simulink model "fig4"  (R2021b)
settings: Solver=VariableStepAuto  StartTime=0.0  StopTime=10.0  RelTol=1e-3
values from neighbouring files (symbols this model uses):
  P = randi(10, [1 length(t)])    [plot_fig8_train_diagram.m]    (also in run_sim_ac.m = fn_get_params_simu(1, N); run_sim_fb1.m = fn_get_params_simu(1, 1); run_sim_fb2.m = P_)
libraries: fuzblock x10
settings Model: Creator=Alex  LastModifiedBy=Alex

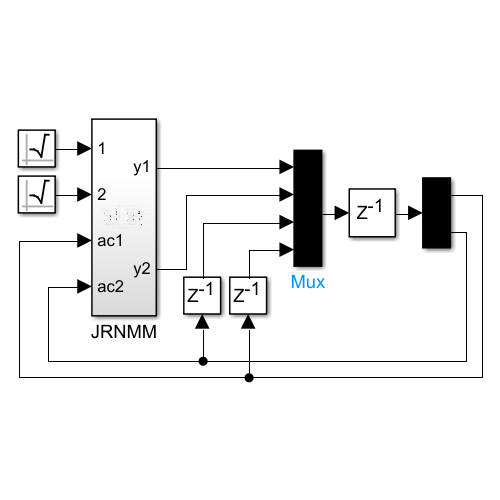
[thumbnail: Simulink's stored preview of the top-level diagram]
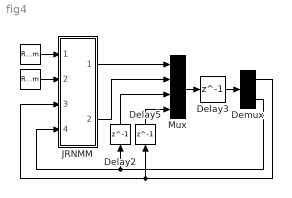
== system fig4 ==
  " " : RandomNumber  Seed=1  SampleTime=0.001
  "  " : RandomNumber  Seed=1  SampleTime=0.001
  Delay2 : Delay  DelayLength=1  InitialCondition=0
  Delay3 : Delay  DelayLength=1  InitialCondition=0
  Delay5 : Delay  DelayLength=1  InitialCondition=0
  Demux : Demux  Outputs=2
  JRNMM : Subsystem
  Mux : Mux
  wires:
  "  "/1 -> JRNMM/1(In2)
  " "/1 -> JRNMM/2(In1)
  JRNMM/1(y1) -> Mux/1
  Demux/1 -> Delay5/1, JRNMM/3(ac1)
  Demux/2 -> JRNMM/4(ac2), Delay2/1
  Mux/1 -> Delay3/1
  Delay3/1 -> Demux/1
  JRNMM/2(y2) -> Mux/2
  Delay2/1 -> Mux/3
  Delay5/1 -> Mux/4

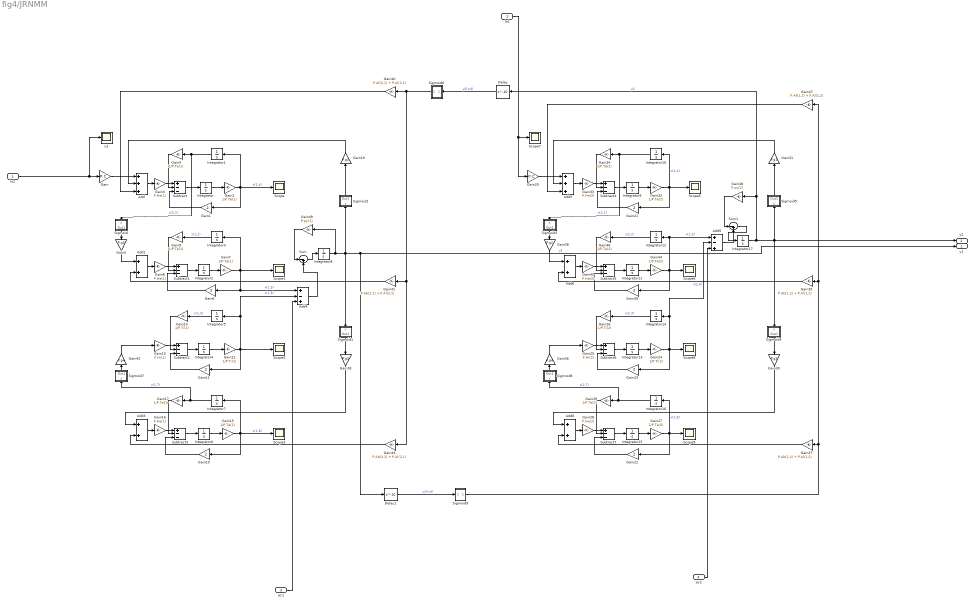
== system fig4/JRNMM ==
  In2 : Inport
  In1 : Inport  Port=2
  ac1 : Inport  Port=3
  ac2 : Inport  Port=4
  Add : Sum  Inputs=+++
  Add{1,3,6,8} (4 alike) : Sum
  Add4 : Sum  Inputs=+-+
  Add5 : Sum  Inputs=+++
  Add9 : Sum  Inputs=+-+
  Delay : Delay  DelayLength=10  InitialCondition=0
  Delay1 : Delay  DelayLength=10  InitialCondition=0  SampleTime=0.-1
  Gain : Gain  Gain=P.C
  Gain{1,6,10..11,21..23,39} (8 alike) : Gain  Gain=2
  Gain12 : Gain  Gain=1/P.Ti(1)
  Gain13 : Gain  Gain=P.Hi(1)
  Gain14 : Gain  Gain=1/P.Ti(1)
  Gain{2,4,7,9,15,17} (6 alike) : Gain  Gain=1/P.Te(1)
  Gain16 : Gain  Gain=P.He(1)
  Gain18 : Gain  Gain=P.g3
  Gain19 : Gain  Gain=P.g1
  Gain20 : Gain  Gain=P.C
  Gain24 : Gain  Gain=1/P.Ti(2)
  Gain25 : Gain  Gain=P.Hi(2)
  Gain26 : Gain  Gain=1/P.Ti(2)
  Gain{27,29,32,34,44,46} (6 alike) : Gain  Gain=1/P.Te(2)
  Gain28 : Gain  Gain=P.He(2)
  Gain3 : Gain  Gain=P.He(1)
  Gain30 : Gain  Gain=P.g3
  Gain31 : Gain  Gain=P.g1
  Gain33 : Gain  Gain=P.He(2)
  Gain35 : Gain  Gain=P.Ab(1,2) + P.Al(1,2)
  Gain36 : Gain  Gain=P.g4
  Gain37 : Gain  Gain=P.Ab(1,2) + P.Al(1,2)
  Gain38 : Gain  Gain=P.g2
  Gain40 : Gain  Gain=P.Af(2,1) + P.Al(2,1)
  Gain41 : Gain  Gain=P.Ab(2,1) + P.Al(2,1)
  Gain42 : Gain  Gain=P.g4
  Gain43 : Gain  Gain=P.Ab(2,1) + P.Al(2,1)
  Gain45 : Gain  Gain=P.He(2)
  Gain47 : Gain  Gain=P.Af(1,2) + P.Al(1,2)
  Gain48 : Gain  Gain=P.py(2)
  Gain49 : Gain  Gain=P.py(1)
  Gain5 : Gain  Gain=P.g2
  Gain8 : Gain  Gain=P.He(1)
  Integrator : Integrator  ContinuousStateAttributes='x14'
  Integrator1 : Integrator  ContinuousStateAttributes='x11'
  Integrator10 : Integrator  ContinuousStateAttributes='x21'
  Integrator11 : Integrator  ContinuousStateAttributes='x25'
  Integrator12 : Integrator  ContinuousStateAttributes='x22'
  Integrator13 : Integrator  ContinuousStateAttributes='x26'
  Integrator14 : Integrator  ContinuousStateAttributes='x23'
  Integrator15 : Integrator  ContinuousStateAttributes='x28'
  Integrator16 : Integrator  ContinuousStateAttributes='x27'
  Integrator17 : Integrator
  Integrator2 : Integrator  ContinuousStateAttributes='x15'
  Integrator3 : Integrator  ContinuousStateAttributes='x12'
  Integrator4 : Integrator  ContinuousStateAttributes='x16'
  Integrator5 : Integrator  ContinuousStateAttributes='x13'
  Integrator6 : Integrator  ContinuousStateAttributes='x18'
  Integrator7 : Integrator  ContinuousStateAttributes='x17'
  Integrator8 : Integrator
  Integrator9 : Integrator  ContinuousStateAttributes='x24'
  Scope{,1..3,5..9} (9 alike) : Scope
  Sigmoid : Subsystem
  Sigmoid1 : Subsystem
  Sigmoid2 : Subsystem
  Sigmoid3 : Subsystem
  Sigmoid4 : Subsystem
  Sigmoid5 : Subsystem
  Sigmoid6 : Subsystem
  Sigmoid7 : Subsystem
  Sigmoid8 : Subsystem
  Sigmoid9 : Subsystem
  Subtract{,1..7} (8 alike) : Sum  Inputs=+--
  Sum : Sum  Inputs=|-+
  Sum1 : Sum  Inputs=|-+
  u1 : Scope
  y1 : Outport
  y2 : Outport  Port=2
  wires:
  Gain34/1 -> Subtract4/2
  Delay/1 -> Sigmoid6/1(x)  "y2(t-d)"
  Gain38/1 -> Add6/1
  Sigmoid6/1(Out1) -> Gain43/1, Gain41/1, Gain40/1
  In2/1 -> u1/1, Gain/1
  Subtract7/1 -> Integrator15/1
  Gain26/1 -> Subtract6/2
  Delay1/1 -> Sigmoid9/1(x)  "y1(t-d)"
  Gain42/1 -> Gain13/1
  Gain2/1 -> Integrator1/1, Scope/1, Gain1/1  "x(1,4)"
  Gain24/1 -> Integrator14/1, Add9/2, Scope8/1, Gain23/1  "x(2,6)"
  Add6/1 -> Gain45/1
  Subtract4/1 -> Integrator9/1
  Add3/1 -> Gain16/1
  Gain39/1 -> Subtract5/3
  Gain19/1 -> Add/2
  Gain7/1 -> Gain6/1, Add4/1, Integrator3/1, Scope1/1  "x(1,5)"
  Integrator13/1 -> Gain24/1
  Subtract1/1 -> Integrator2/1
  Gain35/1 -> Add6/2
  Integrator7/1 -> Sigmoid7/1(x), Gain17/1  "x(1,7)"
  Sigmoid3/1(Out1) -> Gain38/1
  Gain16/1 -> Subtract3/1
  Gain44/1 -> Integrator12/1, Add9/1, Scope6/1, Gain39/1  "x(2,5)"
  Gain43/1 -> Add3/2
  Gain5/1 -> Add1/1
  Integrator9/1 -> Gain32/1
  Integrator3/1 -> Gain9/1  "x(1,2)"
  Gain23/1 -> Subtract6/3
  Integrator10/1 -> Sigmoid3/1(x), Gain34/1  "x(2,1)"
  Sigmoid2/1(Out1) -> Gain19/1
  Gain17/1 -> Subtract3/2
  Gain15/1 -> Integrator7/1, Scope3/1, Gain10/1  "x(1,8)"
  Integrator1/1 -> Sigmoid/1(x), Gain4/1  "x(1,1)"
  Gain41/1 -> Add1/2
  Gain27/1 -> Integrator16/1, Scope9/1, Gain22/1  "x(2,8)"
  Gain14/1 -> Subtract2/2
  Gain1/1 -> Subtract/3
  Integrator14/1 -> Gain26/1  "x(2,3)"
  Gain40/1 -> Add/3
  Gain12/1 -> Integrator5/1, Add4/2, Scope2/1, Gain11/1  "x(1,6)"
  Subtract3/1 -> Integrator6/1
  Integrator11/1 -> Gain44/1
  Gain36/1 -> Gain25/1
  Gain4/1 -> Subtract/2
  Gain46/1 -> Subtract5/2
  Gain32/1 -> Integrator10/1, Scope5/1, Gain21/1  "x(2,4)"
  Gain20/1 -> Add5/1
  Add/1 -> Gain3/1
  In1/1 -> Gain20/1, Scope7/1
  Sigmoid/1(Out1) -> Gain5/1
  Gain9/1 -> Subtract1/2
  Gain/1 -> Add/1
  Sigmoid8/1(Out1) -> Gain36/1
  Integrator4/1 -> Gain12/1
  Add5/1 -> Gain33/1
  Integrator2/1 -> Gain7/1
  Gain18/1 -> Add3/1
  Integrator6/1 -> Gain15/1
  Sigmoid7/1(Out1) -> Gain42/1
  Gain37/1 -> Add8/2
  Gain10/1 -> Subtract3/3
  Integrator8/1 -> Gain49/1, Sigmoid2/1(x), y1/1, Delay1/1, Sigmoid1/1(x)  "y1"
  Sigmoid1/1(Out1) -> Gain18/1
  Integrator16/1 -> Sigmoid8/1(x), Gain29/1  "x(2,7)"
  Integrator17/1 -> y2/1, Sigmoid4/1(x), Sigmoid5/1(x), Delay/1, Gain48/1  "y2"
  Add1/1 -> Gain8/1
  Gain22/1 -> Subtract7/3
  Sigmoid5/1(Out1) -> Gain31/1
  Integrator5/1 -> Gain14/1  "x(1,3)"
  Sigmoid4/1(Out1) -> Gain30/1
  Gain28/1 -> Subtract7/1
  Gain45/1 -> Subtract5/1
  Gain3/1 -> Subtract/1
  Integrator/1 -> Gain2/1
  Integrator12/1 -> Gain46/1  "x(2,2)"
  Subtract2/1 -> Integrator4/1
  Subtract5/1 -> Integrator11/1
  Gain13/1 -> Subtract2/1
  Gain8/1 -> Subtract1/1
  Gain25/1 -> Subtract6/1
  Subtract/1 -> Integrator/1
  Integrator15/1 -> Gain27/1
  Gain6/1 -> Subtract1/3
  Gain11/1 -> Subtract2/3
  Gain21/1 -> Subtract4/3
  Gain31/1 -> Add5/2
  Sigmoid9/1(Out1) -> Gain47/1, Gain35/1, Gain37/1
  Gain47/1 -> Add5/3
  Add8/1 -> Gain28/1
  Gain30/1 -> Add8/1
  Gain29/1 -> Subtract7/2
  Gain33/1 -> Subtract4/1
  Subtract6/1 -> Integrator13/1
  ac1/1 -> Add4/3
  ac2/1 -> Add9/3
  Gain49/1 -> Sum/1
  Add4/1 -> Sum/2
  Sum/1 -> Integrator8/1
  Gain48/1 -> Sum1/1
  Add9/1 -> Sum1/2
  Sum1/1 -> Integrator17/1

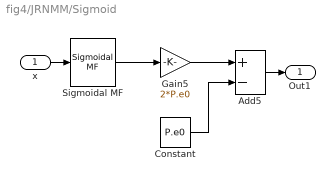
== system fig4/JRNMM/Sigmoid ==
  x : Inport
  Add5 : Sum  Inputs=+-
  Constant : Constant  Value=P.e0
  Gain5 : Gain  Gain=2*P.e0
  Sigmoidal MF : fuzblock/Membership  Functions/Sigmoidal MF  a=P.r  c=P.v0
      settings: SourceProductBaseCode=FL
  Out1 : Outport
  wires:
  Gain5/1 -> Add5/1
  Sigmoidal MF/1 -> Gain5/1
  Constant/1 -> Add5/2
  Add5/1 -> Out1/1
  x/1 -> Sigmoidal MF/1

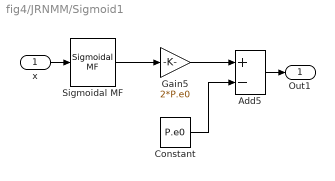
== system fig4/JRNMM/Sigmoid1 ==
  x : Inport
  Add5 : Sum  Inputs=+-
  Constant : Constant  Value=P.e0
  Gain5 : Gain  Gain=2*P.e0
  Sigmoidal MF : fuzblock/Membership  Functions/Sigmoidal MF  a=P.r  c=P.v0
      settings: SourceProductBaseCode=FL
  Out1 : Outport
  wires:
  Gain5/1 -> Add5/1
  Sigmoidal MF/1 -> Gain5/1
  Constant/1 -> Add5/2
  Add5/1 -> Out1/1
  x/1 -> Sigmoidal MF/1

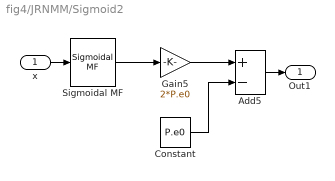
== system fig4/JRNMM/Sigmoid2 ==
  x : Inport
  Add5 : Sum  Inputs=+-
  Constant : Constant  Value=P.e0
  Gain5 : Gain  Gain=2*P.e0
  Sigmoidal MF : fuzblock/Membership  Functions/Sigmoidal MF  a=P.r  c=P.v0
      settings: SourceProductBaseCode=FL
  Out1 : Outport
  wires:
  Gain5/1 -> Add5/1
  Sigmoidal MF/1 -> Gain5/1
  Constant/1 -> Add5/2
  Add5/1 -> Out1/1
  x/1 -> Sigmoidal MF/1

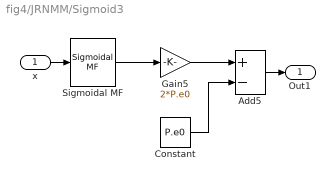
== system fig4/JRNMM/Sigmoid3 ==
  x : Inport
  Add5 : Sum  Inputs=+-
  Constant : Constant  Value=P.e0
  Gain5 : Gain  Gain=2*P.e0
  Sigmoidal MF : fuzblock/Membership  Functions/Sigmoidal MF  a=P.r  c=P.v0
      settings: SourceProductBaseCode=FL
  Out1 : Outport
  wires:
  Gain5/1 -> Add5/1
  Sigmoidal MF/1 -> Gain5/1
  Constant/1 -> Add5/2
  Add5/1 -> Out1/1
  x/1 -> Sigmoidal MF/1

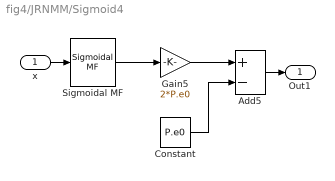
== system fig4/JRNMM/Sigmoid4 ==
  x : Inport
  Add5 : Sum  Inputs=+-
  Constant : Constant  Value=P.e0
  Gain5 : Gain  Gain=2*P.e0
  Sigmoidal MF : fuzblock/Membership  Functions/Sigmoidal MF  a=P.r  c=P.v0
      settings: SourceProductBaseCode=FL
  Out1 : Outport
  wires:
  Gain5/1 -> Add5/1
  Sigmoidal MF/1 -> Gain5/1
  Constant/1 -> Add5/2
  Add5/1 -> Out1/1
  x/1 -> Sigmoidal MF/1

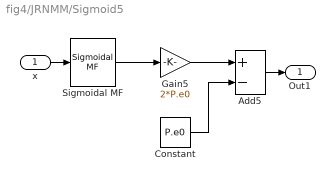
== system fig4/JRNMM/Sigmoid5 ==
  x : Inport
  Add5 : Sum  Inputs=+-
  Constant : Constant  Value=P.e0
  Gain5 : Gain  Gain=2*P.e0
  Sigmoidal MF : fuzblock/Membership  Functions/Sigmoidal MF  a=P.r  c=P.v0
      settings: SourceProductBaseCode=FL
  Out1 : Outport
  wires:
  Gain5/1 -> Add5/1
  Sigmoidal MF/1 -> Gain5/1
  Constant/1 -> Add5/2
  Add5/1 -> Out1/1
  x/1 -> Sigmoidal MF/1

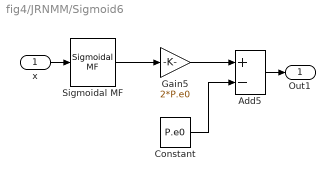
== system fig4/JRNMM/Sigmoid6 ==
  x : Inport
  Add5 : Sum  Inputs=+-
  Constant : Constant  Value=P.e0
  Gain5 : Gain  Gain=2*P.e0
  Sigmoidal MF : fuzblock/Membership  Functions/Sigmoidal MF  a=P.r  c=P.v0
      settings: SourceProductBaseCode=FL
  Out1 : Outport
  wires:
  Gain5/1 -> Add5/1
  Sigmoidal MF/1 -> Gain5/1
  Constant/1 -> Add5/2
  Add5/1 -> Out1/1
  x/1 -> Sigmoidal MF/1

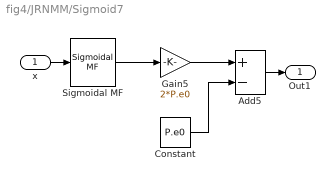
== system fig4/JRNMM/Sigmoid7 ==
  x : Inport
  Add5 : Sum  Inputs=+-
  Constant : Constant  Value=P.e0
  Gain5 : Gain  Gain=2*P.e0
  Sigmoidal MF : fuzblock/Membership  Functions/Sigmoidal MF  a=P.r  c=P.v0
      settings: SourceProductBaseCode=FL
  Out1 : Outport
  wires:
  Gain5/1 -> Add5/1
  Sigmoidal MF/1 -> Gain5/1
  Constant/1 -> Add5/2
  Add5/1 -> Out1/1
  x/1 -> Sigmoidal MF/1

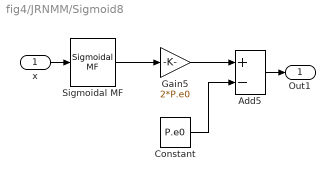
== system fig4/JRNMM/Sigmoid8 ==
  x : Inport
  Add5 : Sum  Inputs=+-
  Constant : Constant  Value=P.e0
  Gain5 : Gain  Gain=2*P.e0
  Sigmoidal MF : fuzblock/Membership  Functions/Sigmoidal MF  a=P.r  c=P.v0
      settings: SourceProductBaseCode=FL
  Out1 : Outport
  wires:
  Gain5/1 -> Add5/1
  Sigmoidal MF/1 -> Gain5/1
  Constant/1 -> Add5/2
  Add5/1 -> Out1/1
  x/1 -> Sigmoidal MF/1

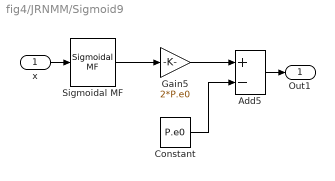
== system fig4/JRNMM/Sigmoid9 ==
  x : Inport
  Add5 : Sum  Inputs=+-
  Constant : Constant  Value=P.e0
  Gain5 : Gain  Gain=2*P.e0
  Sigmoidal MF : fuzblock/Membership  Functions/Sigmoidal MF  a=P.r  c=P.v0
      settings: SourceProductBaseCode=FL
  Out1 : Outport
  wires:
  Gain5/1 -> Add5/1
  Sigmoidal MF/1 -> Gain5/1
  Constant/1 -> Add5/2
  Add5/1 -> Out1/1
  x/1 -> Sigmoidal MF/1
